simulink model "testBCIRobot3e_ext"  (Simulink 7.4)
settings: Solver=FixedStepDiscrete  SolverMode=SingleTasking  StartTime=0.0  StopTime=inf  FixedStep=0.002  MaxStep=0.02  RelTol=1e-3  AbsTol=1e-6
libraries: simulink_extras x1
CloseFcn:
  | rtwprivate ssgencode ModelCloseRequest MC_AD
settings Model: Creator=fwornle  LastModifiedBy=fw  SimulationMode=external  ExtModeTrigDuration=5000  ExtModeLogAll=off
settings ConfigSet: Description=rtmc9s12target_R2009b
settings DataIOCC: LimitDataPoints=off  SaveOutput=off  SaveTime=off  SignalLoggingName=sigsOut
settings OptimizationCC: BlockReduction=off  BooleanDataType=off  InitFltsAndDblsToZero=on  OptimizeModelRefInitCode=on  LifeSpan=1
settings DebuggingCC: SaveWithParameterizedLinksMsg=none  SignalResolutionControl=TryResolveAllWithWarning  SolverPrmCheckMsg=none  MultiTaskDSMMsg=warning  MultiTaskCondExecSysMsg=none  StrictBusMsg=None
settings HardwareCC: ProdBitPerInt=16  ProdEndianess=BigEndian  ProdWordSize=16  ProdHWDeviceType=Motorola HC12
settings RTWCC: SystemTargetFile=mc9s12.tlc  GenerateMakefile=off  TemplateMakefile=mc9s12.tmf  ProcessScript=mc9s12_make_rtw_hook  IncludeERTFirstTime=on
settings CodeAppCC: IgnoreCustomStorageClasses=off
settings STFCustomTargetCC: TargetFcnLib=ansi_tfl_tmw.mat  ModelReferenceCompliant=off  IncludeMdlTerminateFcn=off  ERTCustomFileBanners=on  SupportNonInlinedSFcns=off  CPPClassGenCompliant=on  SystemTargetFile=mc9s12.tlc
settings ERTTargetCC: TargetFcnLib=ansi_tfl_tmw.mat  MultiwordLength=2048  ModelReferenceCompliant=off  ParMdlRefBuildCompliant=off  CompOptLevelCompliant=off  IncludeMdlTerminateFcn=off  CombineOutputUpdateFcns=off  ERTFirstTimeCompliant=off  SupportContinuousTime=on  ModelStepFunctionPrototypeControlCompliant=off  ExtMode=on  ExtModeMexFile=ext_serial_mc9s12_comm  ExtModeMexArgs=1,2,115200  InlinedParameterPlacement=NonHierarchical  ERTCustomFileTemplate=mc9s12_file_process.tlc  GRTInterface=on  ConvertIfToSwitch=off
settings CustomProperty: DataType=RTWOptions_EnumType_C__Users_fw__SVN_rtmc9s12-target_trunk_rtmc9s12_CW_R2009b_bin_mc9s12_1mc9s12_TargetBoard  Value=MiniDragonPlus-RevE
settings EnumStrPairs: String=Dragon12

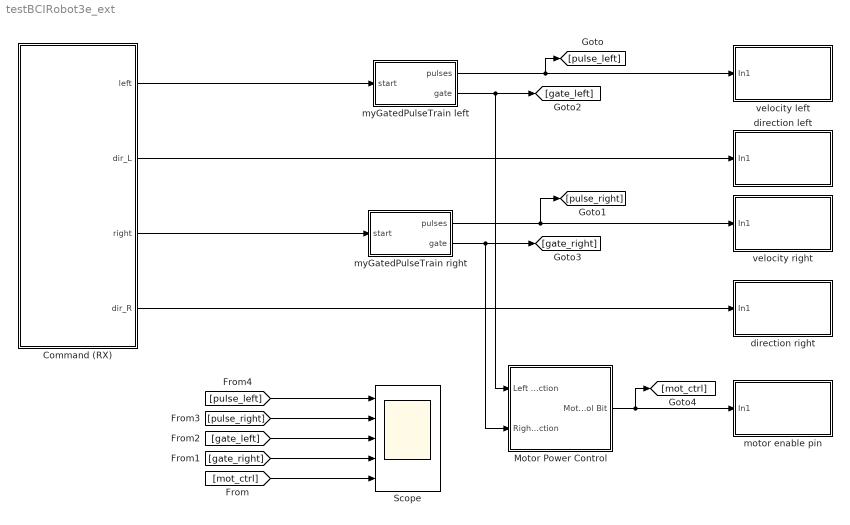
== system testBCIRobot3e_ext ==
  Command (RX) : Subsystem
  Motor Power Control : Subsystem
  Scope : Scope  NumInputPorts=5
      settings: TimeRange=10  YMin=-5~-5~-5~-5~-5  YMax=5~5~5~5~5
  direction left : Subsystem  Tag=mcTarget_digOut  mask{port=Port A, pin=5, sampletime=0.002, Von=0.5, Voff=0.5}
      mask prompts: port "Port (see hardware manuals for valid options)"; pin "Pin (see hardware manuals for valid options)"; sampletime "Sample time"; Von "On-threshold (Von)"; Voff "Off-threshold (Voff)"
      mask init:
      | [portstr, pinstr, pins] = mbc_digitaloutput(port, pin, sampletime, Von, Voff);
      mask Help: web('digOut_sfcn_9S12.html');
      mask StyleString: popup(Port A|Port B|Port H|Port J|Port M|Port P|Port S|Port T),edit,edit,edit,edit
      mask Display: fprintf('%s\nPins: %s', portstr, pinstr)
  direction right : Subsystem  Tag=mcTarget_digOut  mask{port=Port A, pin=7, sampletime=0.002, Von=0.5, Voff=0.5}
      mask prompts: port "Port (see hardware manuals for valid options)"; pin "Pin (see hardware manuals for valid options)"; sampletime "Sample time"; Von "On-threshold (Von)"; Voff "Off-threshold (Voff)"
      mask init:
      | [portstr, pinstr, pins] = mbc_digitaloutput(port, pin, sampletime, Von, Voff);
      mask Help: web('digOut_sfcn_9S12.html');
      mask StyleString: popup(Port A|Port B|Port H|Port J|Port M|Port P|Port S|Port T),edit,edit,edit,edit
      mask Display: fprintf('%s\nPins: %s', portstr, pinstr)
  motor enable pin : Subsystem  Tag=mcTarget_digOut  mask{port=Port T, pin=7, sampletime=0.002, Von=0.5, Voff=0.5}
      mask prompts: port "Port (see hardware manuals for valid options)"; pin "Pin (see hardware manuals for valid options)"; sampletime "Sample time"; Von "On-threshold (Von)"; Voff "Off-threshold (Voff)"
      mask init:
      | [portstr, pinstr, pins] = mbc_digitaloutput(port, pin, sampletime, Von, Voff);
      mask Help: web('digOut_sfcn_9S12.html');
      mask StyleString: popup(Port A|Port B|Port H|Port J|Port M|Port P|Port S|Port T),edit,edit,edit,edit
      mask Display: fprintf('%s\nPins: %s', portstr, pinstr)
  myGatedPulseTrain left : Subsystem  mask{Tcount=0.02, Nsamp=30}
      mask prompts: Tcount "Sample time"; Nsamp "Number of samples"
      mask init:
      | % each period has an on-phase and an off-phase
      | Ncount = 2*Nsamp;
  myGatedPulseTrain right : Subsystem  mask{Tcount=0.02, Nsamp=30}
      mask prompts: Tcount "Sample time"; Nsamp "Number of samples"
      mask init:
      | % each period has an on-phase and an off-phase
      | Ncount = 2*Nsamp;
  velocity left : Subsystem  Tag=mcTarget_digOut  mask{port=Port A, pin=4, sampletime=0.002, Von=0.5, Voff=0.5}
      mask prompts: port "Port (see hardware manuals for valid options)"; pin "Pin (see hardware manuals for valid options)"; sampletime "Sample time"; Von "On-threshold (Von)"; Voff "Off-threshold (Voff)"
      mask init:
      | [portstr, pinstr, pins] = mbc_digitaloutput(port, pin, sampletime, Von, Voff);
      mask Help: web('digOut_sfcn_9S12.html');
      mask StyleString: popup(Port A|Port B|Port H|Port J|Port M|Port P|Port S|Port T),edit,edit,edit,edit
      mask Display: fprintf('%s\nPins: %s', portstr, pinstr)
  velocity right : Subsystem  Tag=mcTarget_digOut  mask{port=Port A, pin=6, sampletime=0.002, Von=0.5, Voff=0.5}
      mask prompts: port "Port (see hardware manuals for valid options)"; pin "Pin (see hardware manuals for valid options)"; sampletime "Sample time"; Von "On-threshold (Von)"; Voff "Off-threshold (Voff)"
      mask init:
      | [portstr, pinstr, pins] = mbc_digitaloutput(port, pin, sampletime, Von, Voff);
      mask Help: web('digOut_sfcn_9S12.html');
      mask StyleString: popup(Port A|Port B|Port H|Port J|Port M|Port P|Port S|Port T),edit,edit,edit,edit
      mask Display: fprintf('%s\nPins: %s', portstr, pinstr)
  wires:
  Motor Power Control/1(Motor Control Bit) -> [mot_ctrl], motor enable pin/1(In1)
  myGatedPulseTrain left/2(gate) -> Motor Power Control/1(Left Motor Instruction), [gate_left]
  myGatedPulseTrain right/2(gate) -> Motor Power Control/2(Right Motor  Instruction), [gate_right]
  myGatedPulseTrain left/1(pulses) -> [pulse_left], velocity left/1(In1)
  myGatedPulseTrain right/1(pulses) -> [pulse_right], velocity right/1(In1)
  Command (RX)/4(dir_R) -> direction right/1(In1)
  Command (RX)/1(left) -> myGatedPulseTrain left/1(start)
  [mot_ctrl] -> Scope/5
  [pulse_left] -> Scope/1
  [pulse_right] -> Scope/2
  [gate_left] -> Scope/3
  [gate_right] -> Scope/4
  Command (RX)/2(dir_L) -> direction left/1(In1)
  Command (RX)/3(right) -> myGatedPulseTrain right/1(start)

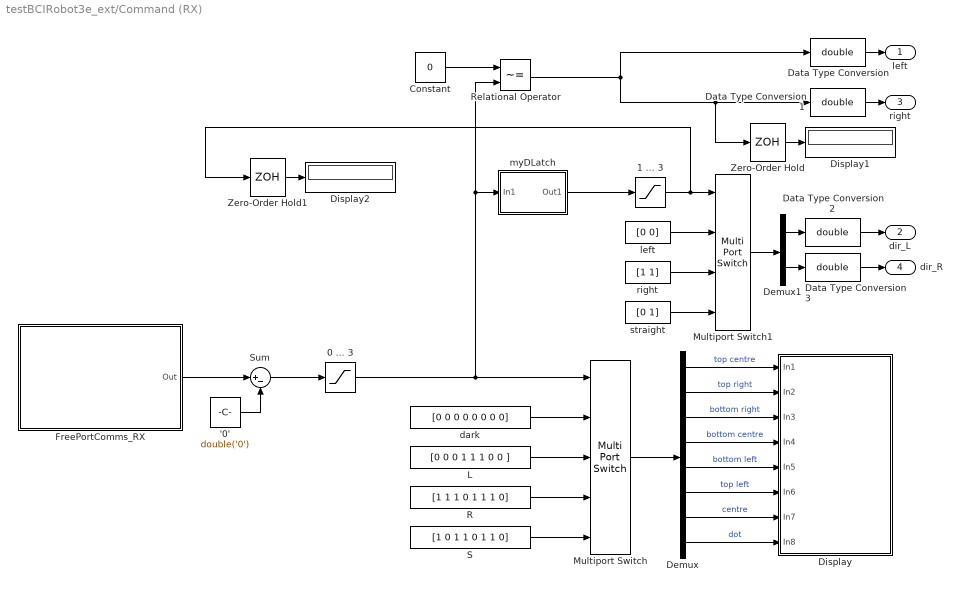
== system testBCIRobot3e_ext/Command (RX) ==
  " left " : Constant  Value=[0 0]  OutDataTypeMode=double  OutDataType=sfix(16)  OutScaling=2^0  OutDataTypeStr=double
  " right " : Constant  Value=[1 1]  OutDataTypeMode=double  OutDataType=sfix(16)  OutScaling=2^0  OutDataTypeStr=double
  " straight " : Constant  Value=[0 1]  OutDataTypeMode=double  OutDataType=sfix(16)  OutScaling=2^0  OutDataTypeStr=double
  '0' : Constant  Value=double('0')  OutDataType=sfix(16)  OutScaling=2^0
  0 ... 3 : Saturate  UpperLimit=3  LowerLimit=0
  1 ... 3 : Saturate  UpperLimit=3  LowerLimit=1
  Constant : Constant  Value=0  OutDataType=sfix(16)  OutScaling=2^0
  Data Type Conversion{,1..3} (4 alike) : DataTypeConversion  OutDataTypeMode=double  OutDataType=sfix(16)  OutScaling=2^0  OutDataTypeStr=double  SaturateOnIntegerOverflow=on  RndMeth=Zero
  Demux : Demux  Outputs=8
  Demux1 : Demux  Outputs=2
  Display : Subsystem  Tag=mcTarget_digOut  mask{port=Port H, pin=0:7, sampletime=0.1, Von=0.5, Voff=0.5}
      mask prompts: port "Port (see hardware manuals for valid options)"; pin "Pin (see hardware manuals for valid options)"; sampletime "Sample time"; Von "On-threshold (Von)"; Voff "Off-threshold (Voff)"
      mask init:
      | [portstr, pinstr, pins] = mbc_digitaloutput(port, pin, sampletime, Von, Voff);
      mask Help: web('digOut_sfcn_9S12.html');
      mask StyleString: popup(Port A|Port B|Port H|Port J|Port M|Port P|Port S|Port T),edit,edit,edit,edit
      mask Display: fprintf('%s\nPins: %s', portstr, pinstr)
  Display1 : Display
  Display2 : Display
  FreePortComms_RX : Subsystem  Tag=mcTarget_freePortCommsRX  mask{sampletime=0.1, port=SCI1, baudrate=115200, channel=0, buf_size=1, data_type=UINT8, format=on, outformat=on}
      mask prompts: sampletime "Sample time"; port "Communication port"; channel "Channel number"; buf_size "Number of elements"; data_type "Data Type"; format "Block receives raw data"; outformat "Block output is double"
      mask init:
      | [buf_sizestr, portNamestr, baudratestr, channelstr, data_type_str, sampletime_str] = mbc_freeportrxd(sampletime, port, baudrate, channel, buf_size, data_type, format, outformat);
      mask Help: web('freePortComms_rxd.html');
      mask StyleString: edit,popup(SCI0|SCI1|COM1|COM2|COM3|COM4),popup(300|600|1200|2400|4800|9600|19200|38400|57600|115200),edit,edit,popup(SINGLE|INT8|UINT8|INT16|UINT16|INT32|UINT32|BOOLEAN),checkbox,checkbox
      mask Display: fprintf('Receive %s element(s)\nComm port: %s\nBaudrate: %s bps\nChannel: %s\nData type: %s\n Sample rate: %s', buf_sizestr, portNamestr, baudratestr, channelstr, data_type_str, sampletime_str)
  L : Constant  Value=[0 0 0 1 1 1 0 0 ]  OutDataTypeMode=double  OutDataType=sfix(16)  OutScaling=2^0  OutDataTypeStr=double
  Multiport Switch : MultiPortSwitch  Inputs=4  zeroidx=on  SaturateOnIntegerOverflow=on
  Multiport Switch1 : MultiPortSwitch  SaturateOnIntegerOverflow=on
  R : Constant  Value=[1 1 1 0 1 1 1 0]  OutDataTypeMode=double  OutDataType=sfix(16)  OutScaling=2^0  OutDataTypeStr=double
  Relational Operator : RelationalOperator  Operator=~=  LogicOutDataTypeMode=Specify via dialog  OutDataTypeStr=uint(8)
  S : Constant  Value=[1 0 1 1 0 1 1 0]  OutDataTypeMode=double  OutDataType=sfix(16)  OutScaling=2^0  OutDataTypeStr=double
  Sum : Sum  Inputs=|+-  OutDataType=sfix(16)  OutScaling=2^0  SaturateOnIntegerOverflow=on
  Zero-Order Hold : ZeroOrderHold  SampleTime=0.1
  Zero-Order Hold1 : ZeroOrderHold  SampleTime=0.1
  dark : Constant  Value=[0 0 0 0 0 0 0 0]  OutDataTypeMode=double  OutDataType=sfix(16)  OutScaling=2^0  OutDataTypeStr=double
  myDLatch : Subsystem
  left : Outport  OutDataType=sfix(16)  OutScaling=2^0
  dir_L : Outport  Port=2  OutDataType=sfix(16)  OutScaling=2^0
  right : Outport  Port=3  OutDataType=sfix(16)  OutScaling=2^0
  dir_R : Outport  Port=4  OutDataType=sfix(16)  OutScaling=2^0
  wires:
  dark/1 -> Multiport Switch/2
  L/1 -> Multiport Switch/3
  R/1 -> Multiport Switch/4
  Constant/1 -> Relational Operator/1
  '0'/1 -> Sum/2
  FreePortComms_RX/1(Out) -> Sum/1
  Demux/1 -> Display/1(In1)  "top centre"
  Demux/2 -> Display/2(In2)  "top right"
  Demux/3 -> Display/3(In3)  "bottom right"
  Demux/4 -> Display/4(In4)  "bottom centre"
  Demux/5 -> Display/5(In5)  "bottom left"
  Demux/6 -> Display/6(In6)  "top left"
  Demux/7 -> Display/7(In7)  "centre"
  Demux/8 -> Display/8(In8)  "dot"
  Multiport Switch/1 -> Demux/1
  S/1 -> Multiport Switch/5
  Data Type Conversion/1 -> left/1
  Data Type Conversion1/1 -> right/1
  " left "/1 -> Multiport Switch1/2
  " right "/1 -> Multiport Switch1/3
  " straight "/1 -> Multiport Switch1/4
  Multiport Switch1/1 -> Demux1/1
  Demux1/1 -> Data Type Conversion2/1
  Demux1/2 -> Data Type Conversion3/1
  1 ... 3/1 -> Multiport Switch1/1, Zero-Order Hold1/1
  Data Type Conversion2/1 -> dir_L/1
  Data Type Conversion3/1 -> dir_R/1
  Relational Operator/1 -> Data Type Conversion/1, Data Type Conversion1/1, Zero-Order Hold/1
  Sum/1 -> 0 ... 3/1
  myDLatch/1(Out1) -> 1 ... 3/1
  Zero-Order Hold/1 -> Display1/1
  Zero-Order Hold1/1 -> Display2/1
  0 ... 3/1 -> myDLatch/1(In1), Relational Operator/2, Multiport Switch/1

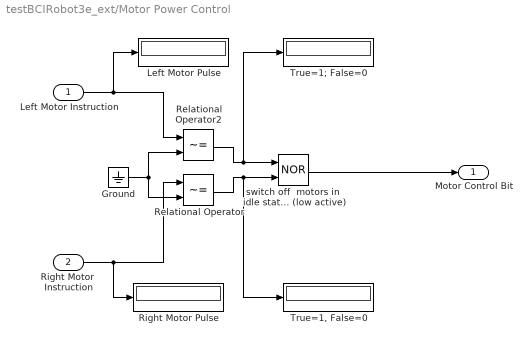
== system testBCIRobot3e_ext/Motor Power Control ==
  Left Motor Instruction : Inport  OutDataType=sfix(16)  OutScaling=2^0
  Right Motor  Instruction : Inport  Port=2  OutDataType=sfix(16)  OutScaling=2^0
  Ground : Ground
  Left Motor Pulse : Display
  Relational Operator : RelationalOperator  Operator=~=
  Relational Operator2 : RelationalOperator  Operator=~=
  Right Motor Pulse : Display
  "True=1, False=0" : Display
  True=1; False=0 : Display
  switch off  motors in  idle state (low active) : Logic  Operator=NOR  AllPortsSameDT=off
  Motor Control Bit : Outport  OutDataType=sfix(16)  OutScaling=2^0
  wires:
  Right Motor  Instruction/1 -> Relational Operator/1, Right Motor Pulse/1
  Left Motor Instruction/1 -> Relational Operator2/1, Left Motor Pulse/1
  Ground/1 -> Relational Operator2/2, Relational Operator/2
  Relational Operator2/1 -> switch off  motors in  idle state (low active)/1, True=1; False=0/1
  Relational Operator/1 -> switch off  motors in  idle state (low active)/2, "True=1, False=0"/1
  switch off  motors in  idle state (low active)/1 -> Motor Control Bit/1

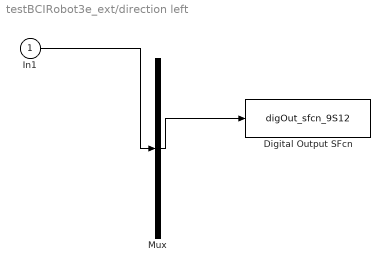
== system testBCIRobot3e_ext/direction left ==
  In1 : Inport  OutDataType=sfix(16)  OutScaling=2^0
  Digital Output SFcn : S-Function  Tag=mcTarget_digOut  FunctionName=digOut_sfcn_9S12  Parameters=sampletime, port, pins, Von, Voff  EnableBusSupport=off
  Mux : Mux  Inputs=1
  wires:
  In1/1 -> Mux/1
  Mux/1 -> Digital Output SFcn/1

== system testBCIRobot3e_ext/direction right ==
  In1 : Inport  OutDataType=sfix(16)  OutScaling=2^0
  Digital Output SFcn : S-Function  Tag=mcTarget_digOut  FunctionName=digOut_sfcn_9S12  Parameters=sampletime, port, pins, Von, Voff  EnableBusSupport=off
  Mux : Mux  Inputs=1
  wires:
  In1/1 -> Mux/1
  Mux/1 -> Digital Output SFcn/1

== system testBCIRobot3e_ext/motor enable pin ==
  In1 : Inport  OutDataType=sfix(16)  OutScaling=2^0
  Digital Output SFcn : S-Function  Tag=mcTarget_digOut  FunctionName=digOut_sfcn_9S12  Parameters=sampletime, port, pins, Von, Voff  EnableBusSupport=off
  Mux : Mux  Inputs=1
  wires:
  In1/1 -> Mux/1
  Mux/1 -> Digital Output SFcn/1

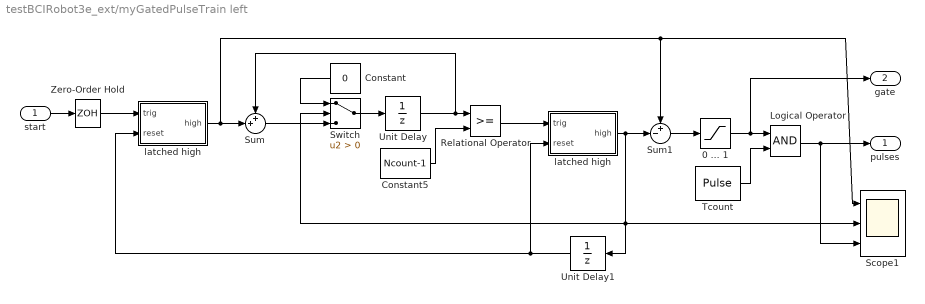
== system testBCIRobot3e_ext/myGatedPulseTrain left ==
  start : Inport  OutDataType=sfix(16)  OutScaling=2^0
  " latched high " : Subsystem
  0 ... 1 : Saturate  UpperLimit=1  LowerLimit=0
  Constant : Constant  Value=0  OutDataType=sfix(16)  OutScaling=2^0
  Constant5 : Constant  Value=Ncount-1  OutDataType=sfix(16)  OutScaling=2^0
  Logical Operator : Logic  AllPortsSameDT=off
  Relational Operator : RelationalOperator  LogicOutDataTypeMode=Specify via dialog  OutDataTypeStr=uint(8)
  Scope1 : Scope  NumInputPorts=3
      settings: YMin=-5~-5~-5  YMax=5~5~5
  Sum : Sum  Inputs=++|  OutDataType=sfix(16)  OutScaling=2^0
  Sum1 : Sum  Inputs=+-|  OutDataType=sfix(16)  OutScaling=2^0
  Switch : Switch  Criteria=u2 > Threshold
  Tcount : DiscretePulseGenerator  Amplitude=1  Period=2  PulseWidth=1  PhaseDelay=0  SampleTime=Tcount
  Unit Delay : UnitDelay  SampleTime=Tcount
  Unit Delay1 : UnitDelay  SampleTime=Tcount
  Zero-Order Hold : ZeroOrderHold  SampleTime=Tcount
  latched high : Subsystem
  pulses : Outport  OutDataType=sfix(16)  OutScaling=2^0
  gate : Outport  Port=2  OutDataType=sfix(16)  OutScaling=2^0
  wires:
  Zero-Order Hold/1 -> latched high/1(trig)
  Logical Operator/1 -> Scope1/3, pulses/1
  Tcount/1 -> Logical Operator/2
  0 ... 1/1 -> gate/1, Logical Operator/1
  Unit Delay1/1 -> latched high/2(reset), " latched high "/2(reset)
  " latched high "/1(high) -> Unit Delay1/1, Switch/2, Scope1/2, Sum1/2
  Relational Operator/1 -> " latched high "/1(trig)
  Sum1/1 -> 0 ... 1/1
  Switch/1 -> Unit Delay/1
  Unit Delay/1 -> Sum/1, Relational Operator/1
  Sum/1 -> Switch/3
  Constant/1 -> Switch/1
  Constant5/1 -> Relational Operator/2
  start/1 -> Zero-Order Hold/1
  latched high/1(high) -> Scope1/1, Sum1/1, Sum/2

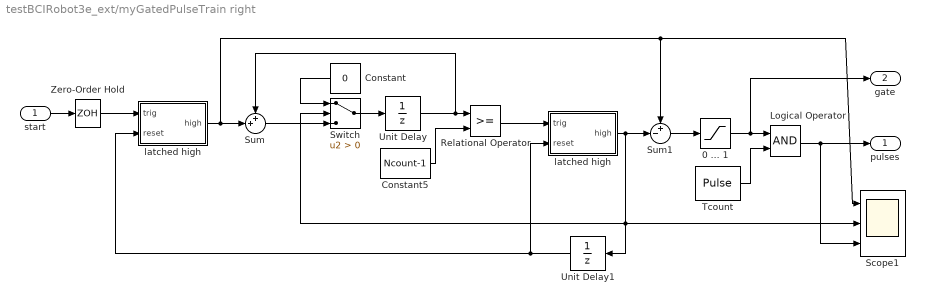
== system testBCIRobot3e_ext/myGatedPulseTrain right ==
  start : Inport  OutDataType=sfix(16)  OutScaling=2^0
  " latched high " : Subsystem
  0 ... 1 : Saturate  UpperLimit=1  LowerLimit=0
  Constant : Constant  Value=0  OutDataType=sfix(16)  OutScaling=2^0
  Constant5 : Constant  Value=Ncount-1  OutDataType=sfix(16)  OutScaling=2^0
  Logical Operator : Logic  AllPortsSameDT=off
  Relational Operator : RelationalOperator  LogicOutDataTypeMode=Specify via dialog  OutDataTypeStr=uint(8)
  Scope1 : Scope  NumInputPorts=3
      settings: YMin=-5~-5~-5  YMax=5~5~5
  Sum : Sum  Inputs=++|  OutDataType=sfix(16)  OutScaling=2^0
  Sum1 : Sum  Inputs=+-|  OutDataType=sfix(16)  OutScaling=2^0
  Switch : Switch  Criteria=u2 > Threshold
  Tcount : DiscretePulseGenerator  Amplitude=1  Period=2  PulseWidth=1  PhaseDelay=0  SampleTime=Tcount
  Unit Delay : UnitDelay  SampleTime=Tcount
  Unit Delay1 : UnitDelay  SampleTime=Tcount
  Zero-Order Hold : ZeroOrderHold  SampleTime=Tcount
  latched high : Subsystem
  pulses : Outport  OutDataType=sfix(16)  OutScaling=2^0
  gate : Outport  Port=2  OutDataType=sfix(16)  OutScaling=2^0
  wires:
  latched high/1(high) -> Sum/2, Sum1/1, Scope1/1
  start/1 -> Zero-Order Hold/1
  Constant5/1 -> Relational Operator/2
  Constant/1 -> Switch/1
  Sum/1 -> Switch/3
  Unit Delay/1 -> Relational Operator/1, Sum/1
  Switch/1 -> Unit Delay/1
  Sum1/1 -> 0 ... 1/1
  Relational Operator/1 -> " latched high "/1(trig)
  " latched high "/1(high) -> Sum1/2, Scope1/2, Switch/2, Unit Delay1/1
  Unit Delay1/1 -> " latched high "/2(reset), latched high/2(reset)
  0 ... 1/1 -> Logical Operator/1, gate/1
  Tcount/1 -> Logical Operator/2
  Logical Operator/1 -> pulses/1, Scope1/3
  Zero-Order Hold/1 -> latched high/1(trig)

== system testBCIRobot3e_ext/velocity left ==
  In1 : Inport  OutDataType=sfix(16)  OutScaling=2^0
  Digital Output SFcn : S-Function  Tag=mcTarget_digOut  FunctionName=digOut_sfcn_9S12  Parameters=sampletime, port, pins, Von, Voff  EnableBusSupport=off
  Mux : Mux  Inputs=1
  wires:
  Mux/1 -> Digital Output SFcn/1
  In1/1 -> Mux/1

== system testBCIRobot3e_ext/velocity right ==
  In1 : Inport  OutDataType=sfix(16)  OutScaling=2^0
  Digital Output SFcn : S-Function  Tag=mcTarget_digOut  FunctionName=digOut_sfcn_9S12  Parameters=sampletime, port, pins, Von, Voff  EnableBusSupport=off
  Mux : Mux  Inputs=1
  wires:
  Mux/1 -> Digital Output SFcn/1
  In1/1 -> Mux/1

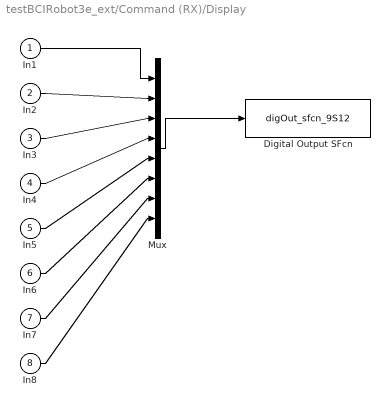
== system testBCIRobot3e_ext/Command (RX)/Display ==
  In1 : Inport  OutDataType=sfix(16)  OutScaling=2^0
  In2 : Inport  Port=2  OutDataType=sfix(16)  OutScaling=2^0
  In3 : Inport  Port=3  OutDataType=sfix(16)  OutScaling=2^0
  In4 : Inport  Port=4  OutDataType=sfix(16)  OutScaling=2^0
  In5 : Inport  Port=5  OutDataType=sfix(16)  OutScaling=2^0
  In6 : Inport  Port=6  OutDataType=sfix(16)  OutScaling=2^0
  In7 : Inport  Port=7  OutDataType=sfix(16)  OutScaling=2^0
  In8 : Inport  Port=8  OutDataType=sfix(16)  OutScaling=2^0
  Digital Output SFcn : S-Function  Tag=mcTarget_digOut  FunctionName=digOut_sfcn_9S12  Parameters=sampletime, port, pins, Von, Voff  EnableBusSupport=off
  Mux : Mux  Inputs=8
  wires:
  In8/1 -> Mux/8
  In7/1 -> Mux/7
  In6/1 -> Mux/6
  In5/1 -> Mux/5
  In4/1 -> Mux/4
  In3/1 -> Mux/3
  In2/1 -> Mux/2
  In1/1 -> Mux/1
  Mux/1 -> Digital Output SFcn/1

== system testBCIRobot3e_ext/Command (RX)/FreePortComms_RX ==
  Data Type Conversion : DataTypeConversion  OutDataTypeMode=double  OutDataType=sfix(16)  OutScaling=2^0  OutDataTypeStr=double  SaturateOnIntegerOverflow=on  RndMeth=Zero
  RECEIVE_FROM_FREE_PORT : S-Function  Tag=mcTarget_freePortCommsRX  FunctionName=freePortComms_rxd  Parameters=sampletime, channel, buf_size, data_type, port, baudrate, format  EnableBusSupport=off
  Out : Outport  OutDataType=sfix(16)  OutScaling=2^0
  wires:
  RECEIVE_FROM_FREE_PORT/1 -> Data Type Conversion/1
  Data Type Conversion/1 -> Out/1

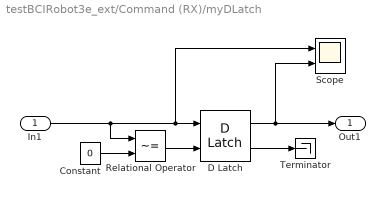
== system testBCIRobot3e_ext/Command (RX)/myDLatch ==
  In1 : Inport  OutDataType=sfix(16)  OutScaling=2^0
  Constant : Constant  Value=0  OutDataType=sfix(16)  OutScaling=2^0
  D Latch : simulink_extras/Flip Flops/D Latch  SystemSampleTime=-1
  Relational Operator : RelationalOperator  Operator=~=
  Scope : Scope  NumInputPorts=2
      settings: YMin=-5~-5  YMax=5~5  SaveName=ScopeData3
  Terminator : Terminator
  Out1 : Outport  OutDataType=sfix(16)  OutScaling=2^0
  wires:
  Relational Operator/1 -> D Latch/2
  Constant/1 -> Relational Operator/2
  In1/1 -> Scope/1, D Latch/1, Relational Operator/1
  D Latch/1 -> Scope/2, Out1/1
  D Latch/2 -> Terminator/1

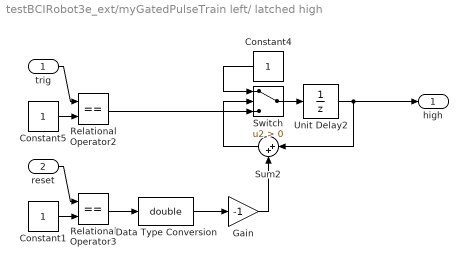
== system testBCIRobot3e_ext/myGatedPulseTrain left/ latched high  ==
  trig : Inport  OutDataType=sfix(16)  OutScaling=2^0
  reset : Inport  Port=2  OutDataType=sfix(16)  OutScaling=2^0
  Constant1 : Constant  OutDataType=sfix(16)  OutScaling=2^0
  Constant4 : Constant  OutDataType=sfix(16)  OutScaling=2^0
  Constant5 : Constant  OutDataType=sfix(16)  OutScaling=2^0
  Data Type Conversion : DataTypeConversion  OutDataTypeMode=double  OutDataType=sfix(16)  OutScaling=2^0  OutDataTypeStr=double  SaturateOnIntegerOverflow=on  RndMeth=Zero
  Gain : Gain  Gain=-1  ParameterDataType=sfix(16)  ParameterScaling=2^0  OutDataType=sfix(16)  OutScaling=2^0  SaturateOnIntegerOverflow=on  OutDataTypeStr=Inherit: Same as input  ParamDataTypeStr=Inherit: Same as input
  Relational Operator2 : RelationalOperator  Operator===  LogicOutDataTypeMode=Specify via dialog  OutDataTypeStr=uint(8)
  Relational Operator3 : RelationalOperator  Operator===  LogicOutDataTypeMode=Specify via dialog  OutDataTypeStr=uint(8)
  Sum2 : Sum  Inputs=|++  OutDataType=sfix(16)  OutScaling=2^0
  Switch : Switch  Criteria=u2 > Threshold
  Unit Delay2 : UnitDelay  SampleTime=-1
  high : Outport  OutDataType=sfix(16)  OutScaling=2^0
  wires:
  trig/1 -> Relational Operator2/1
  reset/1 -> Relational Operator3/1
  Data Type Conversion/1 -> Gain/1
  Gain/1 -> Sum2/2
  Relational Operator3/1 -> Data Type Conversion/1
  Constant1/1 -> Relational Operator3/2
  Sum2/1 -> Switch/2
  Switch/1 -> Unit Delay2/1
  Constant4/1 -> Switch/1
  Unit Delay2/1 -> high/1, Sum2/1
  Relational Operator2/1 -> Switch/3
  Constant5/1 -> Relational Operator2/2

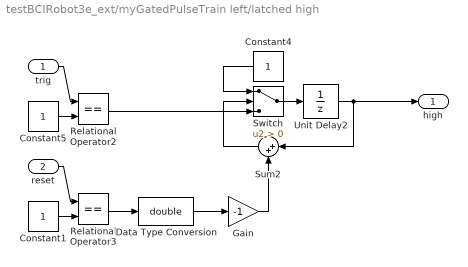
== system testBCIRobot3e_ext/myGatedPulseTrain left/latched high ==
  trig : Inport  OutDataType=sfix(16)  OutScaling=2^0
  reset : Inport  Port=2  OutDataType=sfix(16)  OutScaling=2^0
  Constant1 : Constant  OutDataType=sfix(16)  OutScaling=2^0
  Constant4 : Constant  OutDataType=sfix(16)  OutScaling=2^0
  Constant5 : Constant  OutDataType=sfix(16)  OutScaling=2^0
  Data Type Conversion : DataTypeConversion  OutDataTypeMode=double  OutDataType=sfix(16)  OutScaling=2^0  OutDataTypeStr=double  SaturateOnIntegerOverflow=on  RndMeth=Zero
  Gain : Gain  Gain=-1  ParameterDataType=sfix(16)  ParameterScaling=2^0  OutDataType=sfix(16)  OutScaling=2^0  SaturateOnIntegerOverflow=on  OutDataTypeStr=Inherit: Same as input  ParamDataTypeStr=Inherit: Same as input
  Relational Operator2 : RelationalOperator  Operator===  LogicOutDataTypeMode=Specify via dialog  OutDataTypeStr=uint(8)
  Relational Operator3 : RelationalOperator  Operator===  LogicOutDataTypeMode=Specify via dialog  OutDataTypeStr=uint(8)
  Sum2 : Sum  Inputs=|++  OutDataType=sfix(16)  OutScaling=2^0
  Switch : Switch  Criteria=u2 > Threshold
  Unit Delay2 : UnitDelay  SampleTime=-1
  high : Outport  OutDataType=sfix(16)  OutScaling=2^0
  wires:
  Constant5/1 -> Relational Operator2/2
  Relational Operator2/1 -> Switch/3
  Unit Delay2/1 -> Sum2/1, high/1
  Constant4/1 -> Switch/1
  Switch/1 -> Unit Delay2/1
  Sum2/1 -> Switch/2
  Constant1/1 -> Relational Operator3/2
  Relational Operator3/1 -> Data Type Conversion/1
  Gain/1 -> Sum2/2
  Data Type Conversion/1 -> Gain/1
  reset/1 -> Relational Operator3/1
  trig/1 -> Relational Operator2/1

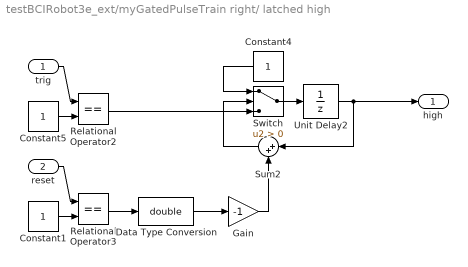
== system testBCIRobot3e_ext/myGatedPulseTrain right/ latched high  ==
  trig : Inport  OutDataType=sfix(16)  OutScaling=2^0
  reset : Inport  Port=2  OutDataType=sfix(16)  OutScaling=2^0
  Constant1 : Constant  OutDataType=sfix(16)  OutScaling=2^0
  Constant4 : Constant  OutDataType=sfix(16)  OutScaling=2^0
  Constant5 : Constant  OutDataType=sfix(16)  OutScaling=2^0
  Data Type Conversion : DataTypeConversion  OutDataTypeMode=double  OutDataType=sfix(16)  OutScaling=2^0  OutDataTypeStr=double  SaturateOnIntegerOverflow=on  RndMeth=Zero
  Gain : Gain  Gain=-1  ParameterDataType=sfix(16)  ParameterScaling=2^0  OutDataType=sfix(16)  OutScaling=2^0  SaturateOnIntegerOverflow=on  OutDataTypeStr=Inherit: Same as input  ParamDataTypeStr=Inherit: Same as input
  Relational Operator2 : RelationalOperator  Operator===  LogicOutDataTypeMode=Specify via dialog  OutDataTypeStr=uint(8)
  Relational Operator3 : RelationalOperator  Operator===  LogicOutDataTypeMode=Specify via dialog  OutDataTypeStr=uint(8)
  Sum2 : Sum  Inputs=|++  OutDataType=sfix(16)  OutScaling=2^0
  Switch : Switch  Criteria=u2 > Threshold
  Unit Delay2 : UnitDelay  SampleTime=-1
  high : Outport  OutDataType=sfix(16)  OutScaling=2^0
  wires:
  Constant5/1 -> Relational Operator2/2
  Relational Operator2/1 -> Switch/3
  Unit Delay2/1 -> Sum2/1, high/1
  Constant4/1 -> Switch/1
  Switch/1 -> Unit Delay2/1
  Sum2/1 -> Switch/2
  Constant1/1 -> Relational Operator3/2
  Relational Operator3/1 -> Data Type Conversion/1
  Gain/1 -> Sum2/2
  Data Type Conversion/1 -> Gain/1
  reset/1 -> Relational Operator3/1
  trig/1 -> Relational Operator2/1

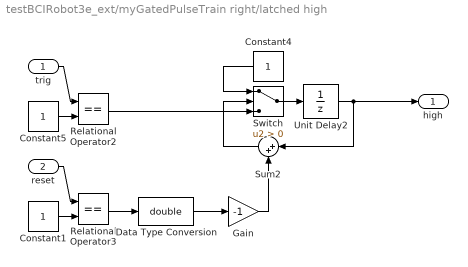
== system testBCIRobot3e_ext/myGatedPulseTrain right/latched high ==
  trig : Inport  OutDataType=sfix(16)  OutScaling=2^0
  reset : Inport  Port=2  OutDataType=sfix(16)  OutScaling=2^0
  Constant1 : Constant  OutDataType=sfix(16)  OutScaling=2^0
  Constant4 : Constant  OutDataType=sfix(16)  OutScaling=2^0
  Constant5 : Constant  OutDataType=sfix(16)  OutScaling=2^0
  Data Type Conversion : DataTypeConversion  OutDataTypeMode=double  OutDataType=sfix(16)  OutScaling=2^0  OutDataTypeStr=double  SaturateOnIntegerOverflow=on  RndMeth=Zero
  Gain : Gain  Gain=-1  ParameterDataType=sfix(16)  ParameterScaling=2^0  OutDataType=sfix(16)  OutScaling=2^0  SaturateOnIntegerOverflow=on  OutDataTypeStr=Inherit: Same as input  ParamDataTypeStr=Inherit: Same as input
  Relational Operator2 : RelationalOperator  Operator===  LogicOutDataTypeMode=Specify via dialog  OutDataTypeStr=uint(8)
  Relational Operator3 : RelationalOperator  Operator===  LogicOutDataTypeMode=Specify via dialog  OutDataTypeStr=uint(8)
  Sum2 : Sum  Inputs=|++  OutDataType=sfix(16)  OutScaling=2^0
  Switch : Switch  Criteria=u2 > Threshold
  Unit Delay2 : UnitDelay  SampleTime=-1
  high : Outport  OutDataType=sfix(16)  OutScaling=2^0
  wires:
  trig/1 -> Relational Operator2/1
  reset/1 -> Relational Operator3/1
  Data Type Conversion/1 -> Gain/1
  Gain/1 -> Sum2/2
  Relational Operator3/1 -> Data Type Conversion/1
  Constant1/1 -> Relational Operator3/2
  Sum2/1 -> Switch/2
  Switch/1 -> Unit Delay2/1
  Constant4/1 -> Switch/1
  Unit Delay2/1 -> high/1, Sum2/1
  Relational Operator2/1 -> Switch/3
  Constant5/1 -> Relational Operator2/2
